simulink model "counter_simulink"  (R2022b)
settings: Solver=FixedStepDiscrete  StartTime=0.0  StopTime=30  FixedStep=1  RelTol=1e-3
settings Model: Creator=Brigosha_Guest  LastModifiedBy=Brigosha_Guest

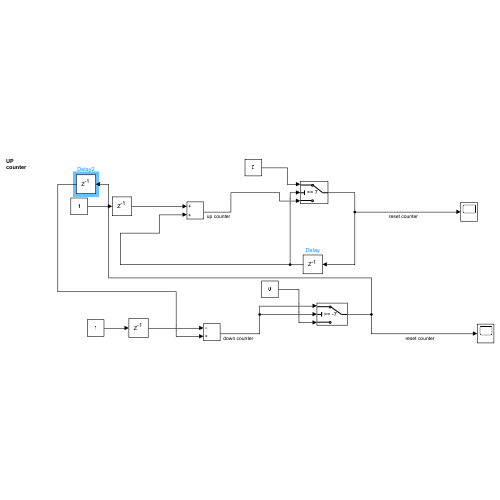
[thumbnail: Simulink's stored preview of the top-level diagram]
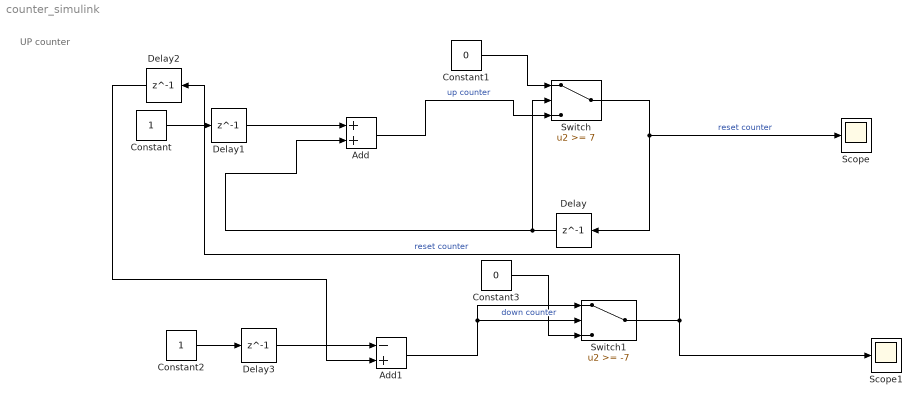
== system counter_simulink ==
  note: UP counter
  Add : Sum
  Add1 : Sum  Inputs=-+
  Constant : Constant
  Constant1 : Constant  Value=0
  Constant2 : Constant
  Constant3 : Constant  Value=0
  Delay{,1..3} (4 alike) : Delay  DelayLength=1
  Scope : Scope
  Scope1 : Scope
  Switch : Switch  Threshold=7  SaturateOnIntegerOverflow=off  InputSameDT=off
  Switch1 : Switch  Threshold=-7  SaturateOnIntegerOverflow=off  InputSameDT=off
  wires:
  Constant/1 -> Delay1/1
  Add/1 -> Switch/3  "up counter"
  Delay/1 -> Switch/2, Add/2
  Delay1/1 -> Add/1
  Constant1/1 -> Switch/1
  Switch/1 -> Delay/1, Scope/1  "reset counter"
  Switch1/1 -> Scope1/1, Delay2/1  "reset counter"
  Constant3/1 -> Switch1/3
  Delay3/1 -> Add1/1
  Delay2/1 -> Add1/2
  Add1/1 -> Switch1/2, Switch1/1  "down counter"
  Constant2/1 -> Delay3/1
